simulink model "cascaded_model"  (R2021a)
settings: Solver=FixedStepAuto  StartTime=0.0  StopTime=30  FixedStep=0.02  RelTol=1e-3
values from neighbouring files (symbols this model uses):
  FF_L = op.inputs(1).u    [trim_boat.m]
  initial_P = op.states(7).x    [trim_boat.m]
  initial_Q = op.states(3).x    [trim_boat.m]
  initial_R = op.states(8).x    [trim_boat.m]
  initial_uspeed = op.states(1).x    [trim_boat.m]
  initial_vspeed = op.states(6).x    [trim_boat.m]
  initial_wspeed = op.states(2).x    [trim_boat.m]
  initial_Z = op.states(5).x    [trim_boat.m]
  rear_alfas = op.inputs(3).u    [trim_boat.m]
  T = op.inputs(4).u    [trim_boat.m]
undefined symbols (not defined in the file or in its folder): ap2, ar2, ay2, bp2, br2, by2, Eff
libraries: simulink x7, pid_lib x1
(part 1 of 2)
settings Model: Creator=Basile  LastModifiedBy=simao
settings SolverCC: ConcurrentTasks=on  ZeroCrossAlgorithm=Adaptive  AlgebraicLoopSolver=TrustRegion  PositivePriorityOrder=on
settings DataIOCC: ExternalInput=getinputstruct(op_trim1)  InitialState=getstatestruct(op_trim1)  SaveOutput=off  DSMLogging=off  SaveTime=off  ReturnWorkspaceOutputs=off
settings OptimizationCC: BlockReduction=off  DefaultParameterBehavior=Inlined  UseDivisionForNetSlopeComputation=on  UseFloatMulNetSlope=on  OptimizeBlockIOStorage=off  BufferReuse=off  PassReuseOutputArgsThreshold=0  EfficientFloat2IntCast=on  OptimizeBlockOrder=speed  DifferentSizesBufferReuse=on
settings DebuggingCC: InheritedTsInSrcMsg=none  ParameterTunabilityLossMsg=error  UnconnectedInputMsg=none  UnconnectedOutputMsg=none  UnconnectedLineMsg=none  UniqueDataStoreMsg=error  SFMachineParentedDataDiag=warning  ArithmeticOperatorsInVariantConditions=warning
settings HardwareCC: ProdBitPerLong=64  ProdLongLongMode=on  ProdHWDeviceType=Intel->x86-64 (Linux 64)
settings SFSimCC: SimUseLocalCustomCode=off  MATLABDynamicMemAlloc=off  CustomCodeUndefinedFunction=UseInterfaceOnly
settings RTWCC: Description=Simulink Real-Time  SystemTargetFile=slrealtime.tlc  TemplateMakefile=slrealtime_default_tmf  GenerateReport=on  RTWUseLocalCustomCode=off  Toolchain=Simulink Real-Time Toolchain  BuildConfiguration=Faster Runs  LaunchReport=on  CodeExecutionProfiling=on  TargetLang=C++
settings CodeAppCC: ForceParamTrailComments=on  OperatorAnnotations=on

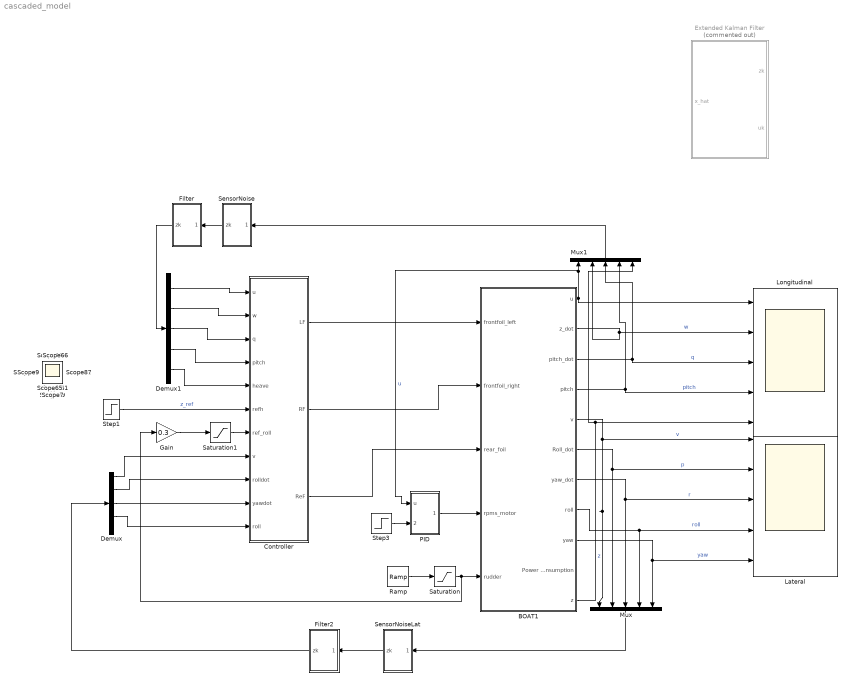
== system cascaded_model ==
  BOAT1 : Subsystem
  Controller : Subsystem
  Demux : Demux  Outputs=5
  Demux1 : Demux  Outputs=5
  Extended Kalman Filter : Subsystem  Commented=on
  Filter : Subsystem
  Filter2 : Subsystem
  Gain : Gain  Gain=0.3
  Lateral : Scope  NumInputPorts=5
  Longitudinal : Scope  NumInputPorts=5
  Mux : Mux  Inputs=5
  Mux1 : Mux  Inputs=5
  PID : Subsystem
  Ramp : simulink/Sources/Ramp  slope=15  start=0  InitialOutput=0
  Saturation : Saturate  UpperLimit=0  LowerLimit=0
  Saturation1 : Saturate  UpperLimit=3  LowerLimit=-3
  SensorNoise : Subsystem
  SensorNoiseLat : Subsystem
  Step1 : Step  Time=20  Before=initial_Z  After=-0.4  SampleTime=0
  Step3 : Step  Time=0  Before=initial_uspeed  After=7  SampleTime=0
  Scope{,1..69} (70 alike) : Scope
  wires:
  BOAT1/2(z_dot) -> Mux1/2, Longitudinal/2  "w"
  BOAT1/3(pitch_dot) -> Mux1/3, Longitudinal/3  "q"
  BOAT1/5(v) -> Mux/1, Lateral/1  "v"
  BOAT1/6(Roll_dot) -> Lateral/2, Mux/2  "p"
  BOAT1/8(roll) -> Lateral/4, Mux/4  "roll"
  BOAT1/11(z) -> Mux1/5, Longitudinal/5  "z"
  BOAT1/1(u) -> Longitudinal/1, PID/1(u), Mux1/1  "u"
  BOAT1/7(yaw_dot) -> Lateral/3, Mux/3  "r"
  Demux1/2 -> Controller/2(w)
  Demux1/3 -> Controller/3(q)
  Demux1/4 -> Controller/4(pitch)
  Demux1/5 -> Controller/5(heave)
  Demux1/1 -> Controller/1(u)
  BOAT1/9(yaw) -> Mux/5, Lateral/5  "yaw"
  BOAT1/4(pitch) -> Mux1/4, Longitudinal/4  "pitch"
  Mux1/1 -> SensorNoise/1(states)
  Mux/1 -> SensorNoiseLat/1(states)
  Step3/1 -> PID/2(In2)
  SensorNoiseLat/1(zk) -> Filter2/1(states)
  Filter/1(zk) -> Demux1/1
  Filter2/1(zk) -> Demux/1
  Ramp/1 -> Saturation/1
  Saturation/1 -> Gain/1, BOAT1/5(rudder)
  Step1/1 -> Controller/6(refh)  "z_ref"
  Demux/1 -> Controller/8(v)
  Demux/2 -> Controller/9(rolldot)
  Demux/3 -> Controller/10(yawdot)
  Demux/4 -> Controller/11(roll)
  Controller/3(ReF) -> BOAT1/3(rear_foil)
  SensorNoise/1(zk) -> Filter/1(states)
  PID/1(rpms_motor) -> BOAT1/4(rpms_motor)
  Gain/1 -> Saturation1/1
  Saturation1/1 -> Controller/7(ref_roll)
  Controller/1(LF) -> BOAT1/1(frontfoil_left)
  Controller/2(RF) -> BOAT1/2(frontfoil_right)

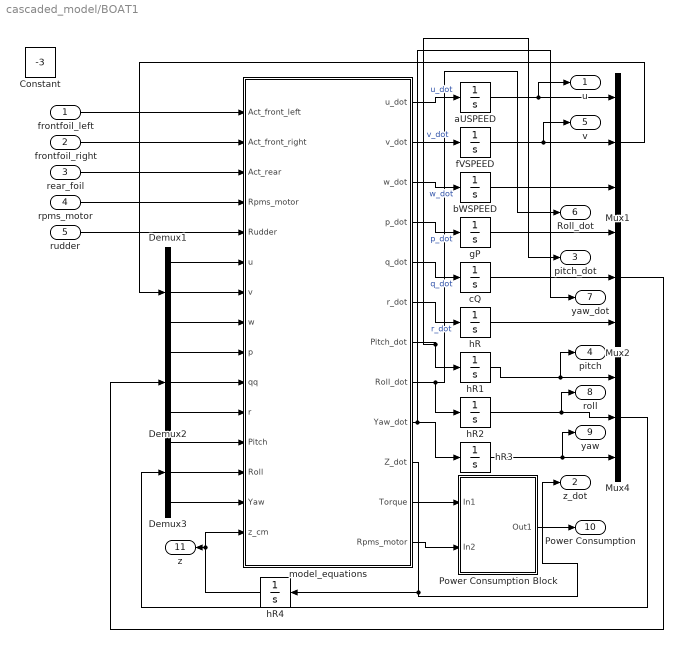
== system cascaded_model/BOAT1 ==
  frontfoil_left : Inport
  frontfoil_right : Inport  Port=2
  rear_foil : Inport  Port=3
  rpms_motor : Inport  Port=4
  rudder : Inport  Port=5
  Constant : Constant  Value=-3
  Demux1 : Demux  Outputs=3
  Demux2 : Demux  Outputs=3
  Demux3 : Demux  Outputs=3
  Mux1 : Mux  Inputs=3
  Mux2 : Mux  Inputs=3
  Mux4 : Mux  Inputs=3
  Power Consumption Block : Subsystem
  aUSPEED : Integrator  InitialCondition=initial_uspeed
  bWSPEED : Integrator  InitialCondition=initial_wspeed
  cQ : Integrator  InitialCondition=initial_Q
  fVSPEED : Integrator  InitialCondition=initial_vspeed
  gP : Integrator  InitialCondition=initial_P
  hR : Integrator  InitialCondition=initial_R
  hR1 : Integrator
  hR2 : Integrator
  hR3 : Integrator
  hR4 : Integrator  InitialCondition=initial_Z
  model_equations : MATLAB Function  TreatAsAtomicUnit=on  VariantControl=Variant1
  u : Outport  VectorParamsAs1DForOutWhenUnconnected=off
  z_dot : Outport  Port=2  VectorParamsAs1DForOutWhenUnconnected=off
  pitch_dot : Outport  Port=3  VectorParamsAs1DForOutWhenUnconnected=off
  pitch : Outport  Port=4  VectorParamsAs1DForOutWhenUnconnected=off
  v : Outport  Port=5  VectorParamsAs1DForOutWhenUnconnected=off
  Roll_dot : Outport  Port=6  VectorParamsAs1DForOutWhenUnconnected=off
  yaw_dot : Outport  Port=7  VectorParamsAs1DForOutWhenUnconnected=off
  roll : Outport  Port=8  VectorParamsAs1DForOutWhenUnconnected=off
  yaw : Outport  Port=9  VectorParamsAs1DForOutWhenUnconnected=off
  Power Consumption : Outport  Port=10  VectorParamsAs1DForOutWhenUnconnected=off
  z : Outport  Port=11  VectorParamsAs1DForOutWhenUnconnected=off
  wires:
  model_equations/6(r_dot) -> hR/1  "r_dot"
  Mux1/1 -> Demux1/1
  model_equations/5(q_dot) -> cQ/1  "q_dot"
  Demux3/2 -> model_equations/13(Roll)
  Demux2/2 -> model_equations/10(qq)
  Demux2/3 -> model_equations/11(r)
  model_equations/4(p_dot) -> gP/1  "p_dot"
  Demux2/1 -> model_equations/9(p)
  rpms_motor/1 -> model_equations/4("Rpms_motor ")
  Demux3/1 -> model_equations/12(Pitch)
  model_equations/2(v_dot) -> fVSPEED/1  "v_dot"
  Demux1/2 -> model_equations/7(v)
  Mux2/1 -> Demux2/1
  Demux3/3 -> model_equations/14(Yaw)
  model_equations/12(Rpms_motor) -> Power Consumption Block/2(In2)
  Power Consumption Block/1(Out1) -> Power Consumption/1
  model_equations/11(Torque) -> Power Consumption Block/1(In1)
  Demux1/1 -> model_equations/6(u)
  cQ/1 -> Mux2/2
  hR/1 -> Mux2/3
  model_equations/3(w_dot) -> bWSPEED/1  "w_dot"
  model_equations/1(u_dot) -> aUSPEED/1  "u_dot"
  gP/1 -> Mux2/1
  model_equations/7(Pitch_dot) -> pitch_dot/1, hR1/1
  model_equations/8(Roll_dot) -> Roll_dot/1, hR2/1
  model_equations/9(Yaw_dot) -> hR3/1, yaw_dot/1
  hR1/1 -> pitch/1, Mux4/1
  hR2/1 -> roll/1, Mux4/2
  hR3/1 -> yaw/1, Mux4/3
  Mux4/1 -> Demux3/1
  rudder/1 -> model_equations/5(Rudder)
  Demux1/3 -> model_equations/8(w)
  fVSPEED/1 -> v/1, Mux1/2
  aUSPEED/1 -> u/1, Mux1/1
  bWSPEED/1 -> Mux1/3
  hR4/1 -> model_equations/15(z_cm), z/1
  frontfoil_left/1 -> model_equations/1(Act_front_left)
  frontfoil_right/1 -> model_equations/2(Act_front_right)
  rear_foil/1 -> model_equations/3(Act_rear)
  model_equations/10(Z_dot) -> hR4/1, z_dot/1

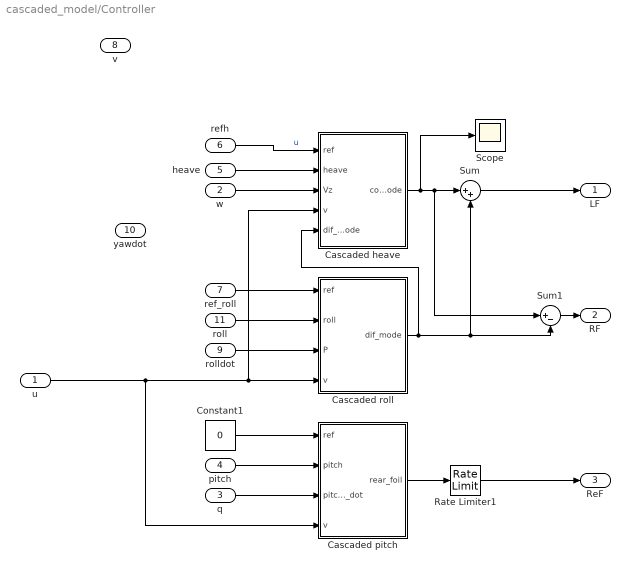
== system cascaded_model/Controller ==
  u : Inport
  w : Inport  Port=2
  q : Inport  Port=3
  pitch : Inport  Port=4
  heave : Inport  Port=5
  refh : Inport  Port=6
  ref_roll : Inport  Port=7
  v : Inport  Port=8
  rolldot : Inport  Port=9
  yawdot : Inport  Port=10
  roll : Inport  Port=11
  Cascaded heave : Subsystem  TreatAsAtomicUnit=on  SystemSampleTime=0.02
  Cascaded pitch : Subsystem  SystemSampleTime=0.02
  Cascaded roll : Subsystem  SystemSampleTime=0.02
  Constant1 : Constant  Value=0
  Rate Limiter1 : RateLimiter  SampleTimeMode=inherited  InitialCondition=rear_alfas
  Scope : Scope
  Sum : Sum  Inputs=|++
  Sum1 : Sum  Inputs=|+-
  LF : Outport  VectorParamsAs1DForOutWhenUnconnected=off
  RF : Outport  Port=2  VectorParamsAs1DForOutWhenUnconnected=off
  ReF : Outport  Port=3  VectorParamsAs1DForOutWhenUnconnected=off
  wires:
  rolldot/1 -> Cascaded roll/3(P)
  roll/1 -> Cascaded roll/2(roll)
  ref_roll/1 -> Cascaded roll/1(ref)
  u/1 -> Cascaded heave/4(v), Cascaded roll/4(v), Cascaded pitch/4(v)
  refh/1 -> Cascaded heave/1(ref)  "u"
  pitch/1 -> Cascaded pitch/2(pitch)
  q/1 -> Cascaded pitch/3(pitch_dot)
  Constant1/1 -> Cascaded pitch/1(ref)
  Cascaded heave/1(com_mode) -> Scope/1, Sum1/1, Sum/1
  Sum/1 -> LF/1
  Cascaded roll/1(dif_mode) -> Cascaded heave/5(dif_mode), Sum1/2, Sum/2
  Sum1/1 -> RF/1
  Rate Limiter1/1 -> ReF/1
  Cascaded pitch/1(rear_foil) -> Rate Limiter1/1
  heave/1 -> Cascaded heave/2(heave)
  w/1 -> Cascaded heave/3(Vz)

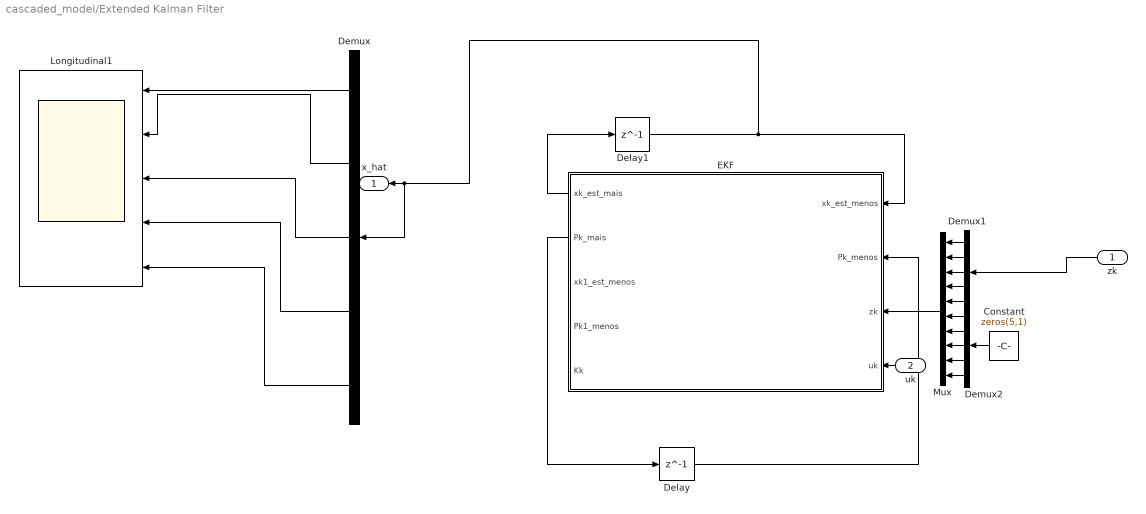
== system cascaded_model/Extended Kalman Filter ==
  zk : Inport  PortDimensions=5
  uk : Inport  Port=2  PortDimensions=5
  Constant : Constant  Value=zeros(5,1)
  Delay : Delay  DelayLength=1  InitialCondition=1000*eye(37)  SampleTime=0.02
  Delay1 : Delay  DelayLength=1  InitialCondition=[initial_uspeed;0;0;0;initial_Z;0;0;0;0;0;zeros(27,1)]  SampleTime=0.02
  Demux : Demux  Outputs=5
  Demux1 : Demux  Outputs=5
  Demux2 : Demux  Outputs=5
  EKF : MATLAB Function  TreatAsAtomicUnit=on
  Longitudinal1 : Scope  NumInputPorts=5
  Mux : Mux  Inputs=10
  x_hat : Outport
  wires:
  uk/1 -> EKF/4(uk)
  Delay/1 -> EKF/2(Pk_menos)
  Demux/1 -> Longitudinal1/1
  Demux/2 -> Longitudinal1/2
  Demux/3 -> Longitudinal1/3
  Demux/4 -> Longitudinal1/4
  Demux/5 -> Longitudinal1/5
  Delay1/1 -> Demux/1, x_hat/1, EKF/1(xk_est_menos)
  EKF/2(Pk_mais) -> Delay/1
  EKF/1(xk_est_mais) -> Delay1/1
  zk/1 -> Demux1/1
  Mux/1 -> EKF/3(zk)
  Demux1/1 -> Mux/1
  Demux1/2 -> Mux/2
  Demux1/3 -> Mux/3
  Demux1/4 -> Mux/4
  Demux1/5 -> Mux/5
  Demux2/1 -> Mux/6
  Demux2/2 -> Mux/7
  Demux2/3 -> Mux/8
  Demux2/4 -> Mux/9
  Demux2/5 -> Mux/10
  Constant/1 -> Demux2/1

== system cascaded_model/Filter ==
  states : Inport
  2nd order Butter : Subsystem
  Demux2 : Demux  Outputs=5
  Longitudinal1 : Scope  NumInputPorts=5
  Mux1 : Mux  Inputs=2
  Mux2 : Mux  Inputs=5
  zk : Outport
  wires:
  states/1 -> Demux2/1
  Mux2/1 -> zk/1
  Demux2/1 -> Mux2/1
  Demux2/2 -> Mux2/2
  Demux2/4 -> Mux2/4
  Demux2/5 -> Mux2/5
  Mux1/1 -> Longitudinal1/3
  2nd order Butter/1(yfilt) -> Mux2/3, Mux1/1
  Demux2/3 -> Mux1/2, 2nd order Butter/1(u)  "q"

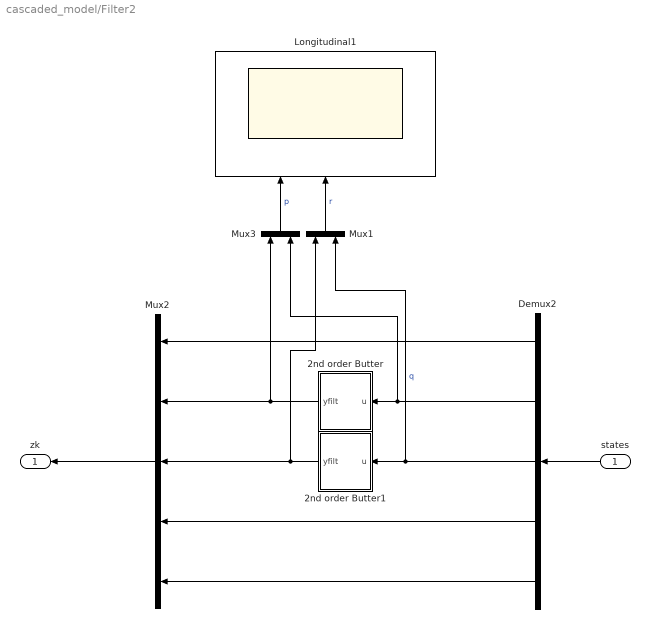
== system cascaded_model/Filter2 ==
  states : Inport
  2nd order Butter : Subsystem
  2nd order Butter1 : Subsystem
  Demux2 : Demux  Outputs=5
  Longitudinal1 : Scope  NumInputPorts=5
  Mux1 : Mux  Inputs=2
  Mux2 : Mux  Inputs=5
  Mux3 : Mux  Inputs=2
  zk : Outport
  wires:
  states/1 -> Demux2/1
  Mux2/1 -> zk/1
  Demux2/1 -> Mux2/1
  Demux2/4 -> Mux2/4
  Demux2/5 -> Mux2/5
  Demux2/2 -> Mux3/2, 2nd order Butter/1(u)
  2nd order Butter1/1(yfilt) -> Mux2/3, Mux1/1
  Demux2/3 -> Mux1/2, 2nd order Butter1/1(u)  "q"
  Mux1/1 -> Longitudinal1/3  "r"
  Mux3/1 -> Longitudinal1/2  "p"
  2nd order Butter/1(yfilt) -> Mux2/2, Mux3/1

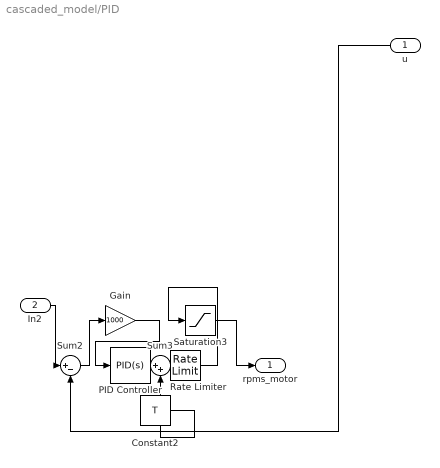
== system cascaded_model/PID ==
  u : Inport
  In2 : Inport  Port=2
  Constant2 : Constant  Value=T
  Gain : Gain  Gain=1000
  PID Controller : pid_lib/PID Controller  Controller=PID  Form=Parallel  TimeDomain=Continuous-time  UseExternalTs=off  SampleTime=-1  IntegratorMethod=Forward Euler  FilterMethod=Forward Euler  ControllerParametersSource=internal  P=1  I=1  D=0.00001  UseFilter=on  N=100  TunerSelectOption=Transfer Function Based (PID Tuner App)  InitialConditionSource=internal  InitialConditionForIntegrator=0  InitialConditionForFilter=0  DifferentiatorICPrevScaledInput=0  ExternalReset=none  TrackingMode=off  Kt=1  LimitOutput=off  SatLimitsSource=internal  UpperSaturationLimit=inf  LowerSaturationLimit=-inf  LinearizeAsGain=on  AntiWindupMode=none  Kb=1  POutMin=[]  POutMax=[]  IOutMin=[]  IOutMax=[]  DOutMin=[]  DOutMax=[]  NOutMin=[]  NOutMax=[]  SumOutMin=[]  SumOutMax=[]  SaturationOutMin=[]  SaturationOutMax=[]  PParamMin=[]  PParamMax=[]  IParamMin=[]  IParamMax=[]  DParamMin=[]  DParamMax=[]  NParamMin=[]  NParamMax=[]  KbParamMin=[]  KbParamMax=[]  KtParamMin=[]  KtParamMax=[]  KbOutMin=[]  KbOutMax=[]  KtOutMin=[]  KtOutMax=[]  IntegratorOutMin=[]  IntegratorOutMax=[]  FilterOutMin=[]  FilterOutMax=[]  SumI1OutMin=[]  SumI1OutMax=[]  SumI2OutMin=[]  SumI2OutMax=[]  SumI3OutMin=[]  SumI3OutMax=[]  SumI4OutMin=[]  SumI4OutMax=[]  SumDOutMin=[]  SumDOutMax=[]  DifferentiatorOutMin=[]  DifferentiatorOutMax=[]  FilterDiffOutCoefMin=[]  FilterDiffOutCoefMax=[]  ReciprocalOutMin=[]  ReciprocalOutMax=[]  SumDenOutMin=[]  SumDenOutMax=[]  SumNumOutMin=[]  SumNumOutMax=[]  DivideOutMin=[]  DivideOutMax=[]  UdiffTsProdOutMin=[]  UdiffTsProdOutMax=[]  NTsProdOutMin=[]  NTsProdOutMax=[]  UintegralTsProdOutMin=[]  UintegralTsProdOutMax=[]  UngainTsProdOutMin=[]  UngainTsProdOutMax=[]  IntegratorContinuousStateAttributes=''  IntegratorStateMustResolveToSignalObject=off  IntegratorRTWStateStorageClass=Auto  FilterContinuousStateAttributes=''  FilterStateMustResolveToSignalObject=off  FilterRTWStateStorageClass=Auto  ParallelPVariant=InternalParameters  IdealPVariant=Disabled  IVariant=InternalParameters  DVariant=InternalParameters  IntegratorVariant=Continuous  SatVariant=Disabled  AWVariant=Passthrough  PCopyVariant=Disabled  TRVariant=Disabled  FdbkBlocksVariant=Forward  IdealPFdbkVariant=Disabled  SatFdbkVariant=Disabled  DerivativeFilterVariant=ContFilter  NVariant=InternalParameters  NCopyVariant=Disabled  FilterICVariant=InternalICsFilter  IntegratorICVariant=InternalICs  ExternalResetVariant=Disabled  TRSumVariant=Passthrough  SumFdbkVariant=Disabled  SumVariant=Sum_PID  TsampFilterVariant=InternalTs  TsampNgainVariant=Passthrough  TsampIntegralVariant=Passthrough  ExternalSaturationOutDataTypeStr=Inherit: Same as second input
  Rate Limiter : RateLimiter  RisingSlewLimit=1000  FallingSlewLimit=-1000  SampleTimeMode=inherited  InitialCondition=T
  Saturation3 : Saturate  UpperLimit=9000
  Sum2 : Sum  Inputs=|+-
  Sum3 : Sum  Inputs=|++
  rpms_motor : Outport
  wires:
  u/1 -> Sum2/2
  Sum3/1 -> Rate Limiter/1
  Gain/1 -> PID Controller/1
  Saturation3/1 -> rpms_motor/1
  PID Controller/1 -> Sum3/1
  Rate Limiter/1 -> Saturation3/1
  Sum2/1 -> Gain/1
  In2/1 -> Sum2/1
  Constant2/1 -> Sum3/2

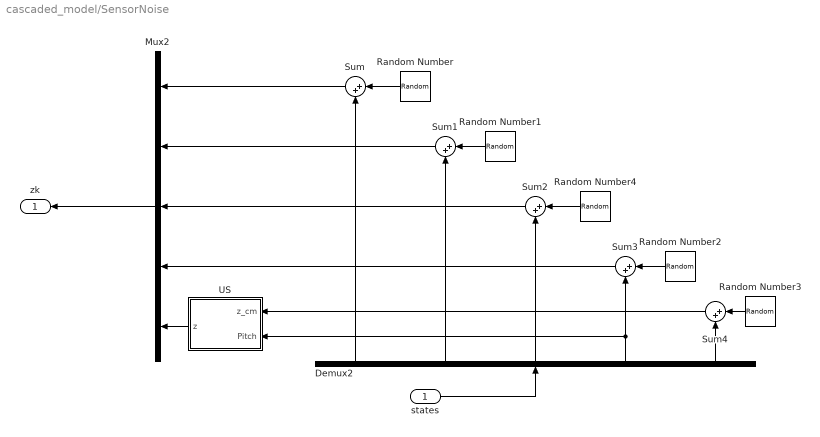
== system cascaded_model/SensorNoise ==
  states : Inport
  Demux2 : Demux  Outputs=5
  Mux2 : Mux  Inputs=5
  Random Number : RandomNumber  Variance=0.001^2  Seed=31233  SampleTime=0.02
  Random Number1 : RandomNumber  Variance=0.001^2  Seed=31232  SampleTime=0.02
  Random Number2 : RandomNumber  Variance=0.005^2  Seed=372323  SampleTime=0.02
  Random Number3 : RandomNumber  Variance=0.0005^2  Seed=312392  SampleTime=0.02
  Random Number4 : RandomNumber  Variance=0.001^2  Seed=31232  SampleTime=0.02
  Sum{,1..4} (5 alike) : Sum  Inputs=|++
  US : MATLAB Function  TreatAsAtomicUnit=on
  zk : Outport
  wires:
  Demux2/1 -> Sum/2
  Demux2/4 -> Sum3/2, US/2(Pitch)
  Demux2/5 -> Sum4/2
  Demux2/2 -> Sum1/2
  states/1 -> Demux2/1
  Mux2/1 -> zk/1
  Sum/1 -> Mux2/1
  Sum3/1 -> Mux2/4
  US/1(z) -> Mux2/5
  Sum4/1 -> US/1(z_cm)
  Sum1/1 -> Mux2/2
  Random Number/1 -> Sum/1
  Random Number3/1 -> Sum4/1
  Random Number2/1 -> Sum3/1
  Sum2/1 -> Mux2/3
  Demux2/3 -> Sum2/2
  Random Number4/1 -> Sum2/1
  Random Number1/1 -> Sum1/1

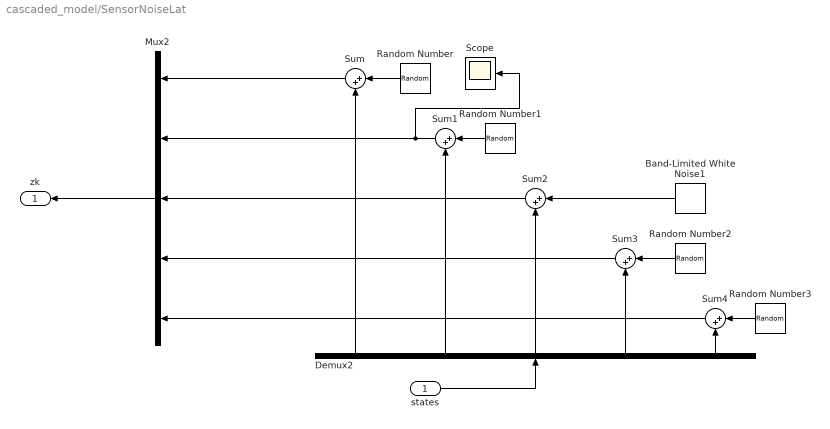
== system cascaded_model/SensorNoiseLat ==
  states : Inport
  Band-Limited White Noise1 : simulink/Sources/Band-Limited White Noise  Cov=[0.0000005]  Ts=0.02  seed=[23341]
  Demux2 : Demux  Outputs=5
  Mux2 : Mux  Inputs=5
  Random Number : RandomNumber  Variance=0.05^2  Seed=31233  SampleTime=0.02
  Random Number1 : RandomNumber  Variance=0.7^2  Seed=372323  SampleTime=0.02
  Random Number2 : RandomNumber  Variance=0.0005^2  Seed=372323  SampleTime=0.02
  Random Number3 : RandomNumber  Variance=0.005^2  Seed=312392  SampleTime=0.02
  Scope : Scope
  Sum{,1..4} (5 alike) : Sum  Inputs=|++
  zk : Outport
  wires:
  Demux2/1 -> Sum/2
  Random Number3/1 -> Sum4/1
  Demux2/4 -> Sum3/2
  Demux2/3 -> Sum2/2
  Demux2/5 -> Sum4/2
  states/1 -> Demux2/1
  Mux2/1 -> zk/1
  Sum/1 -> Mux2/1
  Sum2/1 -> Mux2/3
  Sum3/1 -> Mux2/4
  Sum4/1 -> Mux2/5
  Band-Limited White Noise1/1 -> Sum2/1
  Random Number/1 -> Sum/1
  Demux2/2 -> Sum1/2
  Random Number1/1 -> Sum1/1
  Sum1/1 -> Mux2/2, Scope/1
  Random Number2/1 -> Sum3/1

== system cascaded_model/BOAT1/Power Consumption Block ==
  In1 : Inport
  In2 : Inport  Port=2
  2-D Lookup Table : Lookup_n-D  BreakpointsForDimension1=[1:6000]  BreakpointsForDimension2=[1:140]  Table=Eff  InternalRulePriority=Speed  RndMeth=Simplest  InputSameDT=on
      settings: InputPortMap=u0,u1
  Gain : Gain  Gain=10
  MATLAB Function1 : MATLAB Function  TreatAsAtomicUnit=on
  Out1 : Outport
  wires:
  In2/1 -> 2-D Lookup Table/1, MATLAB Function1/2(Rpms_motor)
  MATLAB Function1/1(P_elec) -> Out1/1
  In1/1 -> Gain/1, MATLAB Function1/1(Torque)
  Gain/1 -> 2-D Lookup Table/2
  2-D Lookup Table/1 -> MATLAB Function1/3(Eficiencia_motor)

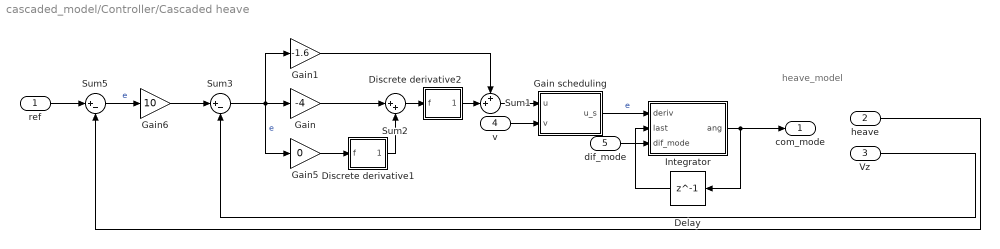
== system cascaded_model/Controller/Cascaded heave ==
  note: heave_model
  ref : Inport
  heave : Inport  Port=2
  Vz : Inport  Port=3
  v : Inport  Port=4
  dif_mode : Inport  Port=5
  Delay : Delay  DelayLength=1  InitialCondition=FF_L  SampleTime=0.02
  Discrete derivative1 : Subsystem
  Discrete derivative2 : Subsystem
  Gain : Gain  Gain=-4
  Gain scheduling : MATLAB Function  TreatAsAtomicUnit=on
  Gain1 : Gain  Gain=-1.6
  Gain5 : Gain  Gain=0
  Gain6 : Gain  Gain=10
  Integrator : MATLAB Function  TreatAsAtomicUnit=on
  Sum1 : Sum  Inputs=++|
  Sum2 : Sum  Inputs=|++
  Sum3 : Sum  Inputs=|+-
  Sum5 : Sum  Inputs=|+-
  com_mode : Outport  VectorParamsAs1DForOutWhenUnconnected=off
  wires:
  Sum3/1 -> Gain5/1, Gain1/1, Gain/1  "e"
  Sum5/1 -> Gain6/1  "e"
  ref/1 -> Sum5/1
  Gain6/1 -> Sum3/1
  Gain/1 -> Sum2/1
  Gain5/1 -> Discrete derivative1/1(f)
  Gain1/1 -> Sum1/1
  Sum2/1 -> Discrete derivative2/1(f)
  Discrete derivative2/1(fdot) -> Sum1/2
  Sum1/1 -> Gain scheduling/1(u)
  Integrator/1(ang) -> com_mode/1, Delay/1
  Delay/1 -> Integrator/2(last)
  Gain scheduling/1(u_s) -> Integrator/1(deriv)  "e"
  heave/1 -> Sum5/2
  Vz/1 -> Sum3/2
  dif_mode/1 -> Integrator/3(dif_mode)
  v/1 -> Gain scheduling/2(v)
  Discrete derivative1/1(fdot) -> Sum2/2

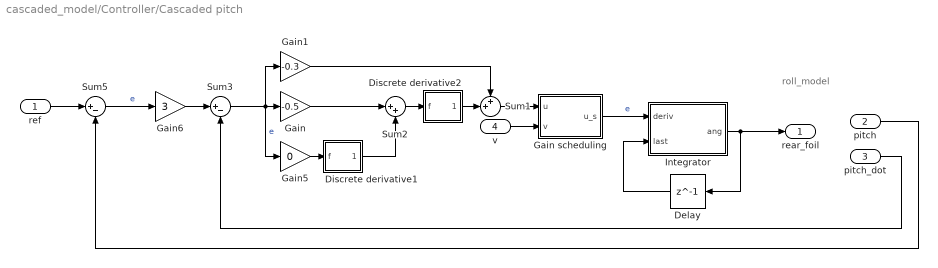
== system cascaded_model/Controller/Cascaded pitch ==
  note: roll_model
  ref : Inport
  pitch : Inport  Port=2
  pitch_dot : Inport  Port=3
  v : Inport  Port=4
  Delay : Delay  DelayLength=1  InitialCondition=rear_alfas  SampleTime=0.02
  Discrete derivative1 : Subsystem
  Discrete derivative2 : Subsystem
  Gain : Gain  Gain=-0.5
  Gain scheduling : MATLAB Function  TreatAsAtomicUnit=on
  Gain1 : Gain  Gain=-0.3
  Gain5 : Gain  Gain=0
  Gain6 : Gain  Gain=3
  Integrator : MATLAB Function  TreatAsAtomicUnit=on
  Sum1 : Sum  Inputs=++|
  Sum2 : Sum  Inputs=|++
  Sum3 : Sum  Inputs=|+-
  Sum5 : Sum  Inputs=|+-
  rear_foil : Outport  VectorParamsAs1DForOutWhenUnconnected=off
  wires:
  Sum3/1 -> Gain5/1, Gain1/1, Gain/1  "e"
  Sum5/1 -> Gain6/1  "e"
  ref/1 -> Sum5/1
  v/1 -> Gain scheduling/2(v)
  Gain6/1 -> Sum3/1
  Gain/1 -> Sum2/1
  pitch/1 -> Sum5/2
  Gain5/1 -> Discrete derivative1/1(f)
  Discrete derivative1/1(fdot) -> Sum2/2
  Gain1/1 -> Sum1/1
  Sum2/1 -> Discrete derivative2/1(f)
  Discrete derivative2/1(fdot) -> Sum1/2
  Sum1/1 -> Gain scheduling/1(u)
  Gain scheduling/1(u_s) -> Integrator/1(deriv)  "e"
  Integrator/1(ang) -> Delay/1, rear_foil/1
  Delay/1 -> Integrator/2(last)
  pitch_dot/1 -> Sum3/2

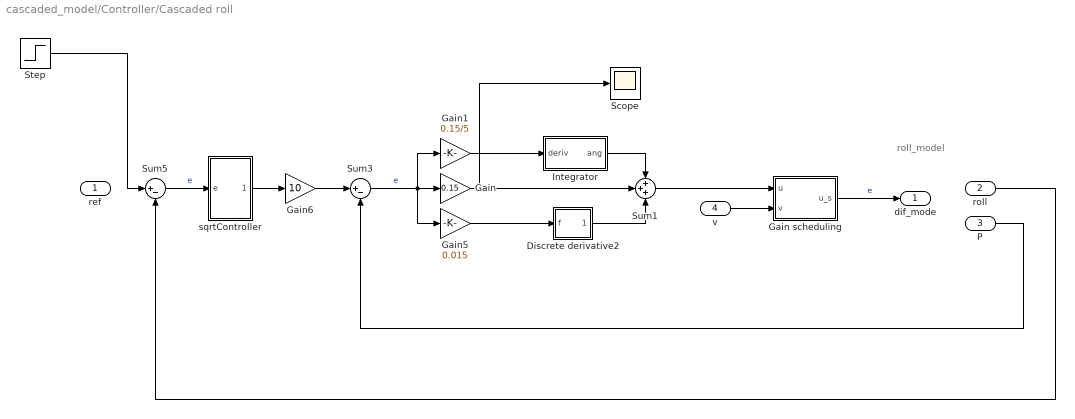
== system cascaded_model/Controller/Cascaded roll ==
  note: roll_model
  ref : Inport
  roll : Inport  Port=2
  P : Inport  Port=3
  v : Inport  Port=4
  Discrete derivative2 : Subsystem
  Gain : Gain  Gain=0.15
  Gain scheduling : MATLAB Function  TreatAsAtomicUnit=on
  Gain1 : Gain  Gain=0.15/5
  Gain5 : Gain  Gain=0.015
  Gain6 : Gain  Gain=10
  Integrator : Subsystem
  Scope : Scope
  Step : Step  Time=0  SampleTime=0
  Sum1 : Sum  Inputs=+++
  Sum3 : Sum  Inputs=|+-
  Sum5 : Sum  Inputs=|+-
  sqrtController : Subsystem
  dif_mode : Outport  VectorParamsAs1DForOutWhenUnconnected=off
  wires:
  v/1 -> Gain scheduling/2(v)
  Gain6/1 -> Sum3/1
  Sum3/1 -> Gain1/1, Gain5/1, Gain/1  "e"
  Gain1/1 -> Integrator/1(deriv)
  Integrator/1(ang) -> Sum1/1
  Gain/1 -> Scope/1, Sum1/2
  Sum1/1 -> Gain scheduling/1(u)
  Gain scheduling/1(u_s) -> dif_mode/1  "e"
  roll/1 -> Sum5/2
  P/1 -> Sum3/2
  Sum5/1 -> sqrtController/1(e)  "e"
  sqrtController/1(Out1) -> Gain6/1
  Step/1 -> Sum5/1
  Gain5/1 -> Discrete derivative2/1(f)
  Discrete derivative2/1(fdot) -> Sum1/3

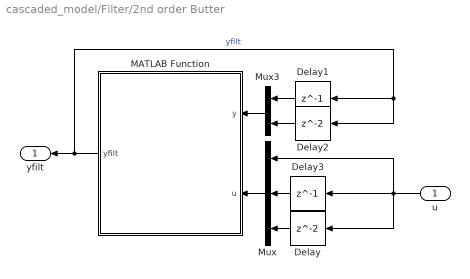
== system cascaded_model/Filter/2nd order Butter ==
  u : Inport
  Delay : Delay
  Delay1 : Delay  DelayLength=1  SampleTime=0.02
  Delay2 : Delay
  Delay3 : Delay  DelayLength=1  SampleTime=0.02
  MATLAB Function : MATLAB Function  TreatAsAtomicUnit=on
  Mux : Mux  Inputs=3
  Mux3 : Mux  Inputs=2
  yfilt : Outport
  wires:
  Mux3/1 -> MATLAB Function/1(y)
  Mux/1 -> MATLAB Function/2(u)
  MATLAB Function/1(yfilt) -> Delay1/1, Delay2/1, yfilt/1  "yfilt"
  Delay/1 -> Mux/3
  Delay3/1 -> Mux/2
  u/1 -> Mux/1, Delay3/1, Delay/1
  Delay1/1 -> Mux3/1
  Delay2/1 -> Mux3/2

== system cascaded_model/Filter2/2nd order Butter ==
  u : Inport
  Delay : Delay
  Delay1 : Delay  DelayLength=1  SampleTime=0.02
  Delay2 : Delay
  Delay3 : Delay  DelayLength=1  SampleTime=0.02
  MATLAB Function : MATLAB Function  TreatAsAtomicUnit=on
  Mux : Mux  Inputs=3
  Mux3 : Mux  Inputs=2
  yfilt : Outport
  wires:
  Mux3/1 -> MATLAB Function/1(y)
  Mux/1 -> MATLAB Function/2(u)
  MATLAB Function/1(yfilt) -> Delay1/1, Delay2/1, yfilt/1  "yfilt"
  Delay/1 -> Mux/3
  Delay3/1 -> Mux/2
  u/1 -> Mux/1, Delay3/1, Delay/1
  Delay1/1 -> Mux3/1
  Delay2/1 -> Mux3/2

== system cascaded_model/Filter2/2nd order Butter1 ==
  u : Inport
  Delay : Delay
  Delay1 : Delay  DelayLength=1  SampleTime=0.02
  Delay2 : Delay
  Delay3 : Delay  DelayLength=1  SampleTime=0.02
  MATLAB Function : MATLAB Function  TreatAsAtomicUnit=on
  Mux : Mux  Inputs=3
  Mux3 : Mux  Inputs=2
  yfilt : Outport
  wires:
  Mux3/1 -> MATLAB Function/1(y)
  Mux/1 -> MATLAB Function/2(u)
  MATLAB Function/1(yfilt) -> Delay1/1, Delay2/1, yfilt/1  "yfilt"
  Delay/1 -> Mux/3
  Delay3/1 -> Mux/2
  u/1 -> Mux/1, Delay3/1, Delay/1
  Delay1/1 -> Mux3/1
  Delay2/1 -> Mux3/2

== system cascaded_model/Controller/Cascaded heave/Discrete derivative1 ==
  f : Inport
  Constant : Constant  Value=0
  Discrete Derivative : simulink/Discrete/Discrete Derivative  gainval=1.0  ICPrevScaledInput=0.0  OutMin=[]  OutMax=[]  OutDataType=fixdt(1, 16)  OutScaling=2^-10  DoSatur=off
  Step : Step  Time=0.01  Before=-1
  Switch : Switch  Criteria=u2 > Threshold
  fdot : Outport  VectorParamsAs1DForOutWhenUnconnected=off
  wires:
  Discrete Derivative/1 -> Switch/1  "ddtkz"
  Constant/1 -> Switch/3
  Step/1 -> Switch/2
  f/1 -> Discrete Derivative/1
  Switch/1 -> fdot/1

== system cascaded_model/Controller/Cascaded heave/Discrete derivative2 ==
  f : Inport
  Constant : Constant  Value=0
  Discrete Derivative : simulink/Discrete/Discrete Derivative  gainval=1.0  ICPrevScaledInput=0.0  OutMin=[]  OutMax=[]  OutDataType=fixdt(1, 16)  OutScaling=2^-10  DoSatur=off
  Step : Step  Time=0.01  Before=-1
  Switch : Switch  Criteria=u2 > Threshold
  fdot : Outport  VectorParamsAs1DForOutWhenUnconnected=off
  wires:
  Discrete Derivative/1 -> Switch/1  "ddtkz"
  Constant/1 -> Switch/3
  Step/1 -> Switch/2
  f/1 -> Discrete Derivative/1
  Switch/1 -> fdot/1

== system cascaded_model/Controller/Cascaded pitch/Discrete derivative1 ==
  f : Inport
  Constant : Constant  Value=0
  Discrete Derivative : simulink/Discrete/Discrete Derivative  gainval=1.0  ICPrevScaledInput=0.0  OutMin=[]  OutMax=[]  OutDataType=fixdt(1, 16)  OutScaling=2^-10  DoSatur=off
  Step : Step  Time=0.01  Before=-1
  Switch : Switch  Criteria=u2 > Threshold
  fdot : Outport  VectorParamsAs1DForOutWhenUnconnected=off
  wires:
  Discrete Derivative/1 -> Switch/1  "ddtkz"
  Constant/1 -> Switch/3
  Step/1 -> Switch/2
  f/1 -> Discrete Derivative/1
  Switch/1 -> fdot/1

== system cascaded_model/Controller/Cascaded pitch/Discrete derivative2 ==
  f : Inport
  Constant : Constant  Value=0
  Discrete Derivative : simulink/Discrete/Discrete Derivative  gainval=1.0  ICPrevScaledInput=0.0  OutMin=[]  OutMax=[]  OutDataType=fixdt(1, 16)  OutScaling=2^-10  DoSatur=off
  Step : Step  Time=0.01  Before=-1
  Switch : Switch  Criteria=u2 > Threshold
  fdot : Outport  VectorParamsAs1DForOutWhenUnconnected=off
  wires:
  Discrete Derivative/1 -> Switch/1  "ddtkz"
  Constant/1 -> Switch/3
  Step/1 -> Switch/2
  f/1 -> Discrete Derivative/1
  Switch/1 -> fdot/1

== system cascaded_model/Controller/Cascaded roll/Discrete derivative2 ==
  f : Inport
  Constant : Constant  Value=0
  Discrete Derivative : simulink/Discrete/Discrete Derivative  gainval=1.0  ICPrevScaledInput=0.0  OutMin=[]  OutMax=[]  OutDataType=fixdt(1, 16)  OutScaling=2^-10  DoSatur=off
  Step : Step  Time=0.01  Before=-1
  Switch : Switch  Criteria=u2 > Threshold
  fdot : Outport  VectorParamsAs1DForOutWhenUnconnected=off
  wires:
  Discrete Derivative/1 -> Switch/1  "ddtkz"
  Constant/1 -> Switch/3
  Step/1 -> Switch/2
  f/1 -> Discrete Derivative/1
  Switch/1 -> fdot/1

== system cascaded_model/Controller/Cascaded roll/Integrator ==
  deriv : Inport
  Delay1 : Delay  DelayLength=1  InitialCondition=0  SampleTime=0.02
  Integrator : MATLAB Function  TreatAsAtomicUnit=on
  ang : Outport
  wires:
  Delay1/1 -> Integrator/2(last)
  Integrator/1(ang) -> ang/1, Delay1/1
  deriv/1 -> Integrator/1(deriv)

== system cascaded_model/Controller/Cascaded roll/sqrtController ==
  e : Inport
  Abs : Abs
  Product : Product
  Sign : Signum
  Sqrt : Sqrt  SaturateOnIntegerOverflow=on
  Out1 : Outport
  wires:
  Product/1 -> Out1/1
  e/1 -> Sign/1, Abs/1
  Abs/1 -> Sqrt/1
  Sqrt/1 -> Product/2
  Sign/1 -> Product/1

== matlab function cascaded_model/Controller/Cascaded heave/Gain scheduling ==
  data: u input; u_s output; v input
function u_s = fcn(u,v)
v_ref = 7;
if(v>v_ref)
    u_s = u*v_ref^2/v^2;
else
    u_s = u;
end

== matlab function cascaded_model/SensorNoise/US ==
  data: z_cm input; z output; Pitch input
function z = fcn(z_cm,Pitch)
Roll = 0; %Approximation
dist_cm_Us_x = 3.150;   %distance between cm and US
z = (z_cm*cosd(Roll)-tand(Pitch)*dist_cm_Us_x)/cosd(Pitch);

== matlab function cascaded_model/Controller/Cascaded roll/Gain scheduling ==
  data: u input; u_s output; v input
function u_s = fcn(u,v)
v_ref = 7;
if(v>v_ref)
    u_s = u*v_ref^2/v^2;
else
    u_s = u;
end

== matlab function cascaded_model/Filter/2nd order Butter/MATLAB Function ==
  data: y input; u input; yfilt output; bp2 parameter; ap2 parameter
function yfilt = filtit(y,u, bp2, ap2)
b = bp2;
a = ap2;
yfilt = 0;
for i=1:length(u)
   yfilt = yfilt + b(i)*u(i);
end

for i=2:length(y)+1
   yfilt = yfilt - a(i)*y(i-1); 
end

yfilt = yfilt/a(1);

end

== matlab function cascaded_model/Controller/Cascaded roll/Integrator/Integrator ==
  data: deriv input; last input; ang output
function ang = fcn(deriv, last)

%% Slew rate limit
max_rate = 10; %º/s
if deriv > max_rate
    deriv = max_rate;
elseif deriv < -max_rate
    deriv = -max_rate;
end

ang = last + deriv*0.02;

%% Ang limit
upper_lim = 8.5;
lower_lim = -8.5;

if ang > upper_lim 
    ang = upper_lim;
elseif ang < lower_lim
    ang = lower_lim;
end

== matlab function cascaded_model/Filter2/2nd order Butter/MATLAB Function ==
  data: y input; u input; yfilt output; br2 parameter; ar2 parameter
function yfilt = filtit(y,u, br2, ar2)
b = br2;
a = ar2;
yfilt = 0;
for i=1:length(u)
   yfilt = yfilt + b(i)*u(i);
end

for i=2:length(y)+1
   yfilt = yfilt - a(i)*y(i-1); 
end

yfilt = yfilt/a(1);

end

== matlab function cascaded_model/Extended Kalman Filter/EKF ==
  data: xk_est_mais output; xk_est_menos input; Pk_menos input; zk input; Pk_mais output; xk1_est_menos output; Pk1_menos output; Kk output; uk input
function [xk_est_mais,Pk_mais,xk1_est_menos,Pk1_menos,Kk] = extended_kalman_filter(xk_est_menos,Pk_menos,zk,uk)

%EKF matrices
Rk = diag([0.05^2 0.05^2 0.25^2 0.25^2 0.005^2 0 0 0 0 0]); 
Qku = eye(10); %Quando tiver erro de modelo

%% RKM Aproximation

%Prediction Phase
%Phik = Jacobian_func_out(xk_est_menos(1),xk_est_menos(2),xk_est_menos(3),xk_est_menos(4),xk_est_menos(5),xk_est_menos(6),xk_est_menos(7),xk_est_menos(8),xk_est_menos(9),uk(3),uk(2),uk(1),uk(4),uk(5));
Phik = fwjac(xk,uk);
Phik = expm(Phik*0.02);
Qk = Phik*Qku*Phik'*0.02;
xk1_est_menos = RKM_EKF(xk_est_menos,uk);
Pk1_menos = Phik*Pk_menos*Phik'+Qk;

%Correction Phase
yk = xk1_est_menos;
Hk = Hk_func(xk1_est_menos(4),xk1_est_menos(5),xk1_est_menos(9));
yk(5) = (yk(5)*cosd(yk(9))-tand(yk(4))*dist_cm_Us_x)/cosd(yk(4)); 
Kk = Pk1_menos*Hk'*inv(Hk*Pk1_menos*Hk'+Rk);
xk_est_mais = xk1_est_menos+Kk*(zk-yk);
Pk_mais = (eye(10)-Kk*Hk)*Pk1_menos*(eye(10)-Kk*Hk)'+Kk*Rk*Kk';
end

== matlab function cascaded_model/BOAT1/Power Consumption Block/MATLAB Function1 ==
  data: Torque input; P_elec output; Rpms_motor input; Eficiencia_motor input
function P_elec = fcn(Torque,Rpms_motor,Eficiencia_motor)
P_mec = Torque*Rpms_motor*2*pi/60;
P_elec = P_mec/Eficiencia_motor;
